simulink model "ENV_old"  (R2024b)
settings: Solver=FixedStepDiscrete  StartTime=0.0  StopTime=1  FixedStep=0.001  RelTol=1e-3  EnableMultiTasking=on
libraries: stm32blockslib x84, canmsglib x40, stm32f4xxblockslib x8, simulink x7
(part 2 of 4)

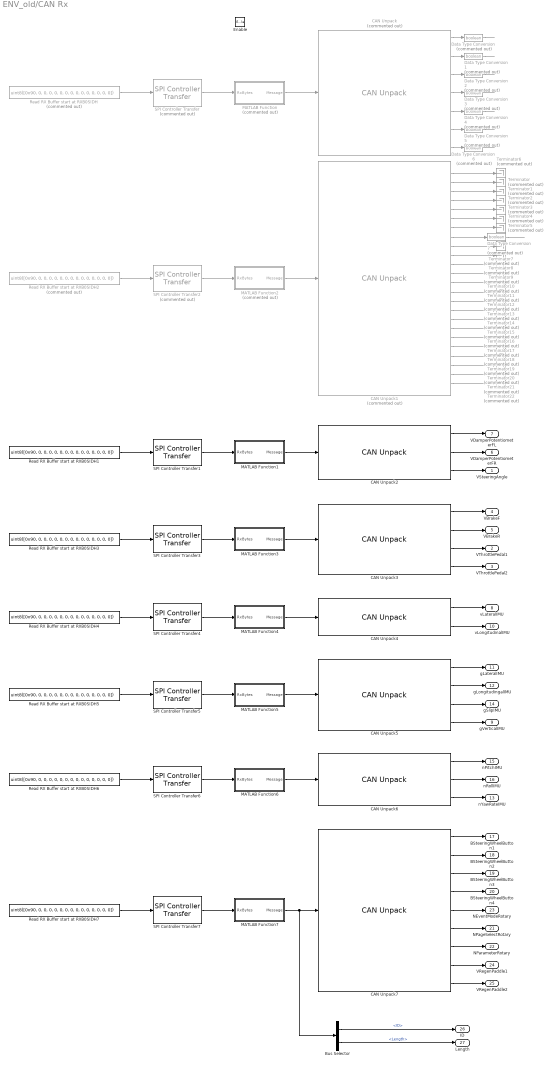
== system ENV_old/CAN Rx ==
  Enable : EnablePort
  Bus Selector : BusSelector  OutputSignals=ID,Length
  CAN Unpack : canmsglib/CAN Unpack  Commented=on  CANdbFile=C:\Users\oxbro\Documents\STM32CustomProjects\PDUSTM32\CAN3_28.06.26.dbc  MsgList=VCU_PDMReq  MsgName=VCU_PDMReq  MsgIDType=Standard (11-bit identifier)  MsgIdentifier=1539  MsgLength=7  SignalInfo={'BAccuFanOn','24','8','LE','unsigned','Standard','0','1','0','0','255';'BBrakeLight','0','8','LE','unsigned','Standard','0','1','0','0','255';'BInvLVOn','32','8','LE','unsigned','Standard','0','1','0','0','255';'BInverterFanOn','8','8','LE','unsigned','Standard','0','1','0','0','255';'BMotorRBHFanOn','16','8','LE','unsigned','Standard','0','8','0','0','255';'BPCComplete','40','8','LE','unsigned','Standard','0','1','0','0','255';'BReadyToDriveBuzzer','48','8','LE','unsigned','Standard','0','1','0','0','255'}  IDPort=off  TimestampPort=off  ErrorPort=off  RemotePort=off  LengthPort=off  StatusPort=off  ApplyMinMax=off
      settings: LibrarySourceBlock=stmutilitieslib/CAN Unpack  DataFormat=CANdb specified signals
  CAN Unpack1 : canmsglib/CAN Unpack  Commented=on  CANdbFile=C:\Users\will\Desktop\STM32Projects\PDUSTM32\CAN3_28.06.26.dbc  MsgList=VCU_1s_Frame4  MsgName=VCU_1s_Frame4  MsgIDType=Standard (11-bit identifier)  MsgIdentifier=419  MsgLength=6  SignalInfo={'BBMSP0A0COut','32','1','LE','unsigned','Standard','0','1','0','0','1';'BBMSP0A0EOut','33','1','LE','unsigned','Standard','0','1','0','0','1';'BBMSP0A10Out','34','1','LE','unsigned','Standard','0','1','0','0','1';'BBMSP0A80Out','35','1','LE','unsigned','Standard','0','1','0','0','1';'BBMSP0AC0Out','36','1','LE','unsigned','Standard','0','1','0','0','1';'BBMSP0AFAOut','37','1','LE','unsigned','Standard','0','1','0','0','1';'BBalancingOnOut','31','1','LE','unsigned','Standard','0','1','0','0','1';'BDrivetrainCoolingOn','1','1','LE','unsigned','Standard','0','1','0','0','1';'BDrivetrainCoolingOnEM','5','1','LE','unsigned','Standard','0','1','0','0','1';'BDrivetrainCoolingOnOW','6','2','LE','unsigned','Standard','0','1','-1','-1','2';'BEMSOn','13','1','LE','unsigned','Standard','0','1','0','0','1';'BEMSOnEM','14','1','LE','unsigned','Standard','0','1','0','0','1';'BEMSOnOW','15','2','LE','unsigned','Standard','0','1','-1','-1','2';'BSpinningModeOn','17','1','LE','unsigned','Standard','0','1','0','0','1';'BSpinningModeOnEM','18','1','LE','unsigned','Standard','0','1','0','0','1';'BSpinningModeOnOW','19','2','LE','unsigned','Standard','0','1','-1','-1','2';'BTCOn','9','1','LE','unsigned','Standard','0','1','0','0','1';'BTCOnEM','10','1','LE','unsigned','Standard','0','1','0','0','1';'BTCOnOW','11','2','LE','unsigned','Standard','0','1','-1','-1','2';'BTVOnEM','0','1','LE','unsigned','Standard','0','1','0','0','1';'BTVOnOW','2','2','LE','unsigned','Standard','0','1','-1','-1','2';'NEventMode','44','4','LE','unsigned','Standard','0','1','0','0','15';'NLap','38','6','LE','unsigned','Standard','0','1','0','0','63';'rSoE','21','10','LE','unsigned','Standard','0','0.1','0','0','102.3'}  IDPort=off  TimestampPort=off  ErrorPort=off  RemotePort=off  LengthPort=off  StatusPort=off  ApplyMinMax=off
      settings: LibrarySourceBlock=stmutilitieslib/CAN Unpack  DataFormat=CANdb specified signals
  CAN Unpack2 : canmsglib/CAN Unpack  CANdbFile=C:\Users\oxbro\Documents\STM32CustomProjects\VCUSTM32\OBR26_Controls_30-7-26\CAN\CAN3\CAN3_03.08.26.dbc  MsgList=DDU7_SteerDamper  MsgName=DDU7_SteerDamper  MsgIDType=Standard (11-bit identifier)  MsgIdentifier=257  MsgLength=8  SignalInfo={'VDamperPotentiometerFL','16','13','LE','unsigned','Standard','0','1','0','0','8191';'VDamperPotentiometerFR','29','13','LE','unsigned','Standard','0','1','0','0','8191';'VSteeringAngle','0','13','LE','unsigned','Standard','0','1','0','0','8191'}  IDPort=off  TimestampPort=off  ErrorPort=off  RemotePort=off  LengthPort=off  StatusPort=off  ApplyMinMax=off
      settings: LibrarySourceBlock=stmutilitieslib/CAN Unpack  DataFormat=CANdb specified signals
  CAN Unpack3 : canmsglib/CAN Unpack  CANdbFile=C:\Users\oxbro\Documents\STM32CustomProjects\VCUSTM32\OBR26_Controls_30-7-26\CAN\CAN3\CAN3_03.08.26.dbc  MsgList=DDU7_ThrBrake  MsgName=DDU7_ThrBrake  MsgIDType=Standard (11-bit identifier)  MsgIdentifier=256  MsgLength=8  SignalInfo={'VBrakeF','0','16','LE','unsigned','Standard','0','1','0','0','3276.75';'VBrakeR','16','16','LE','unsigned','Standard','0','1','0','0','65535';'VThrottlePedal1','32','16','LE','unsigned','Standard','0','1','0','0','65535';'VThrottlePedal2','48','16','LE','unsigned','Standard','0','1','0','0','65535'}  IDPort=off  TimestampPort=off  ErrorPort=off  RemotePort=off  LengthPort=off  StatusPort=off  ApplyMinMax=off
      settings: LibrarySourceBlock=stmutilitieslib/CAN Unpack  DataFormat=CANdb specified signals
  CAN Unpack4 : canmsglib/CAN Unpack  CANdbFile=C:\Users\oxbro\Documents\STM32CustomProjects\VCUSTM32\OBR26_Controls_30-7-26\CAN\CAN3\CAN3_03.08.26.dbc  MsgList=IMU_0x604  MsgName=IMU_0x604  MsgIDType=Standard (11-bit identifier)  MsgIdentifier=1540  MsgLength=8  SignalInfo={'vLateralIMU','16','16','LE','signed','Standard','0','0.01','0','-327.68','327.67';'vLongitudinalIMU','0','16','LE','signed','Standard','0','0.01','0','-327.68','327.67'}  IDPort=off  TimestampPort=off  ErrorPort=off  RemotePort=off  LengthPort=off  StatusPort=off  ApplyMinMax=off
      settings: LibrarySourceBlock=stmutilitieslib/CAN Unpack  DataFormat=CANdb specified signals
  CAN Unpack5 : canmsglib/CAN Unpack  CANdbFile=C:\Users\oxbro\Documents\STM32CustomProjects\VCUSTM32\OBR26_Controls_30-7-26\CAN\CAN3\CAN3_03.08.26.dbc  MsgList=IMU_0x606  MsgName=IMU_0x606  MsgIDType=Standard (11-bit identifier)  MsgIdentifier=1542  MsgLength=8  SignalInfo={'gLateralIMU','16','16','LE','signed','Standard','0','0.01','0','-327.68','327.67';'gLongitudinalIMU','0','16','LE','signed','Standard','0','0.01','0','-327.68','327.67';'gSlipIMU','48','16','LE','signed','Standard','0','0.01','0','-327.68','327.67';'gVerticalIMU','32','16','LE','signed','Standard','0','0.01','0','-327.68','327.67'}  IDPort=off  TimestampPort=off  ErrorPort=off  RemotePort=off  LengthPort=off  StatusPort=off  ApplyMinMax=off
      settings: LibrarySourceBlock=stmutilitieslib/CAN Unpack  DataFormat=CANdb specified signals
  CAN Unpack6 : canmsglib/CAN Unpack  CANdbFile=C:\Users\oxbro\Documents\STM32CustomProjects\VCUSTM32\OBR26_Controls_30-7-26\CAN\CAN3\CAN3_03.08.26.dbc  MsgList=IMU_0x609  MsgName=IMU_0x609  MsgIDType=Standard (11-bit identifier)  MsgIdentifier=1545  MsgLength=8  SignalInfo={'nPitchIMU','16','16','LE','signed','Standard','0','0.01','0','-327.68','327.67';'nRollIMU','0','16','LE','signed','Standard','0','0.01','0','-327.68','327.67';'nYawRateIMU','32','16','LE','signed','Standard','0','0.01','0','-327.68','327.67'}  IDPort=off  TimestampPort=off  ErrorPort=off  RemotePort=off  LengthPort=off  StatusPort=off  ApplyMinMax=off
      settings: LibrarySourceBlock=stmutilitieslib/CAN Unpack  DataFormat=CANdb specified signals
  CAN Unpack7 : canmsglib/CAN Unpack  CANdbFile=C:\Users\oxbro\Documents\STM32CustomProjects\VCUSTM32\OBR26_Controls_30-7-26\CAN\CAN3\CAN3_03.08.26.dbc  MsgList=STW_0x1FB  MsgName=STW_0x1FB  MsgIDType=Standard (11-bit identifier)  MsgIdentifier=507  MsgLength=6  SignalInfo={'BSteeringWheelButton1','0','1','LE','unsigned','Standard','0','1','0','0','1';'BSteeringWheelButton2','1','1','LE','unsigned','Standard','0','1','0','0','1';'BSteeringWheelButton3','2','1','LE','unsigned','Standard','0','1','0','0','1';'BSteeringWheelButton4','3','1','LE','unsigned','Standard','0','1','0','0','1';'NEventModeRotary','20','8','LE','unsigned','Standard','0','1','1','1','16';'NPageSelectRotary','4','8','LE','unsigned','Standard','0','1','1','1','16';'NParameterRotary','12','8','LE','unsigned','Standard','0','1','1','1','16';'VRegenPaddle1','28','8','LE','unsigned','Standard','0','0.0129','0','0','3.2895';'VRegenPaddle2','36','8','LE','unsigned','Standard','0','0.0129','0','0','3.2895'}  IDPort=off  TimestampPort=off  ErrorPort=off  RemotePort=off  LengthPort=off  StatusPort=off  ApplyMinMax=off
      settings: LibrarySourceBlock=stmutilitieslib/CAN Unpack  DataFormat=CANdb specified signals
  Data Type Conversion{,1..7} (8 alike) : DataTypeConversion  Commented=on  OutDataTypeStr=boolean  SaturateOnIntegerOverflow=off  RndMeth=Floor
  MATLAB Function : MATLAB Function  Commented=on  TreatAsAtomicUnit=on
  MATLAB Function1 : MATLAB Function  TreatAsAtomicUnit=on
  MATLAB Function2 : MATLAB Function  Commented=on  TreatAsAtomicUnit=on
  MATLAB Function3 : MATLAB Function  TreatAsAtomicUnit=on
  MATLAB Function4 : MATLAB Function  TreatAsAtomicUnit=on
  MATLAB Function5 : MATLAB Function  TreatAsAtomicUnit=on
  MATLAB Function6 : MATLAB Function  TreatAsAtomicUnit=on
  MATLAB Function7 : MATLAB Function  TreatAsAtomicUnit=on
  Read RX Buffer start at RXB0SIDH : Constant  Commented=on  Value=uint8([0x90, 0, 0, 0, 0, 0, 0, 0, 0, 0, 0, 0, 0, 0, 0])
  Read RX Buffer start at RXB0SIDH{1,3..7} (6 alike) : Constant  Value=uint8([0x90, 0, 0, 0, 0, 0, 0, 0, 0, 0, 0, 0, 0, 0, 0])
  Read RX Buffer start at RXB0SIDH2 : Constant  Commented=on  Value=uint8([0x90, 0, 0, 0, 0, 0, 0, 0, 0, 0, 0, 0, 0, 0, 0])
  SPI Controller Transfer : stm32blockslib/SPI Controller Transfer  Priority=1  Commented=on  SPIModuleSelect=SPI1  ClockPolarity=Low  ClockPhase=1 Edge  SPIModule=uint32(0)  Mode=Master  BusSpeed=uint32(1000000)  FirstBitToTransfer=Most significant bit (MSB)  ClockMode=0  BlockFunction=Transfer  EnableRegisterAddress=off  RegisterAddress=0  OutputDataType=uint8  OutputDataLength=1  OutputStatus=off  BlockingMode=on  Timeout=0.01  DataBits=8  UseCustomSSPin=Explicit GPIO calls  ActiveLowSSPin=Active low  Port_Select=GPIOA  Pin=1
      settings: LibrarySourceBlock=stm32h7xxblockslib/SPI Controller Transfer
  SPI Controller Transfer{1,3..7} (6 alike) : stm32blockslib/SPI Controller Transfer  Priority=1  SPIModuleSelect=SPI1  ClockPolarity=Low  ClockPhase=1 Edge  SPIModule=uint32(0)  Mode=Master  BusSpeed=uint32(1000000)  FirstBitToTransfer=Most significant bit (MSB)  ClockMode=0  BlockFunction=Transfer  EnableRegisterAddress=off  RegisterAddress=0  OutputDataType=uint8  OutputDataLength=1  OutputStatus=off  BlockingMode=on  Timeout=0.01  DataBits=8  UseCustomSSPin=Explicit GPIO calls  ActiveLowSSPin=Active low  Port_Select=GPIOA  Pin=1
      settings: LibrarySourceBlock=stm32h7xxblockslib/SPI Controller Transfer
  SPI Controller Transfer2 : stm32blockslib/SPI Controller Transfer  Priority=1  Commented=on  SPIModuleSelect=SPI1  ClockPolarity=Low  ClockPhase=1 Edge  SPIModule=uint32(0)  Mode=Master  BusSpeed=uint32(1000000)  FirstBitToTransfer=Most significant bit (MSB)  ClockMode=0  BlockFunction=Transfer  EnableRegisterAddress=off  RegisterAddress=0  OutputDataType=uint8  OutputDataLength=1  OutputStatus=off  BlockingMode=on  Timeout=0.01  DataBits=8  UseCustomSSPin=Explicit GPIO calls  ActiveLowSSPin=Active low  Port_Select=GPIOA  Pin=1
      settings: LibrarySourceBlock=stm32h7xxblockslib/SPI Controller Transfer
  Terminator{,1..22} (23 alike) : Terminator  Commented=on
  VSteeringAngle : Outport  OutDataTypeStr=double
  VThrottlePedal1 : Outport  Port=2  OutDataTypeStr=double
  VThrottlePedal2 : Outport  Port=3  OutDataTypeStr=double
  VBrakeF : Outport  Port=4  OutDataTypeStr=double
  VBrakeR : Outport  Port=5  OutDataTypeStr=double
  VDamperPotentiometerFR : Outport  Port=6  OutDataTypeStr=double
  VDamperPotentiometerFL : Outport  Port=7  OutDataTypeStr=double
  vLateralIMU : Outport  Port=8  OutDataTypeStr=double
  gVerticalIMU : Outport  Port=9  OutDataTypeStr=double
  vLongitudinalIMU : Outport  Port=10  OutDataTypeStr=double
  gLateralIMU : Outport  Port=11  OutDataTypeStr=double
  gLongitudingalIMU : Outport  Port=12  OutDataTypeStr=double
  nYawRateIMU : Outport  Port=13  OutDataTypeStr=double
  gSlipIMU : Outport  Port=14  OutDataTypeStr=double
  nPitchIMU : Outport  Port=15  OutDataTypeStr=double
  nRollIMU : Outport  Port=16  OutDataTypeStr=double
  BSteeringWheelButton1 : Outport  Port=17  OutDataTypeStr=boolean
  BSteeringWheelButton2 : Outport  Port=18  OutDataTypeStr=boolean
  BSteeringWheelButton3 : Outport  Port=19  OutDataTypeStr=boolean
  BSteeringWheelButton4 : Outport  Port=20  OutDataTypeStr=boolean
  NPageSelectRotary : Outport  Port=21  OutDataTypeStr=double
  NParameterRotary : Outport  Port=22  OutDataTypeStr=double
  NEventModeRotary : Outport  Port=23  OutDataTypeStr=double
  VRegenPaddle1 : Outport  Port=24  OutDataTypeStr=double
  VRegenPaddle2 : Outport  Port=25  OutDataTypeStr=double
  ID : Outport  Port=26
  Length : Outport  Port=27
  wires:
  Read RX Buffer start at RXB0SIDH/1 -> SPI Controller Transfer/1
  SPI Controller Transfer/1 -> MATLAB Function/1(RxBytes)
  MATLAB Function/1(Message) -> CAN Unpack/1
  CAN Unpack/1 -> Data Type Conversion/1
  CAN Unpack/2 -> Data Type Conversion1/1
  CAN Unpack1/2 -> Terminator/1
  CAN Unpack1/3 -> Terminator1/1
  CAN Unpack1/4 -> Terminator2/1
  CAN Unpack1/5 -> Terminator3/1
  CAN Unpack1/6 -> Terminator4/1
  CAN Unpack1/7 -> Terminator5/1
  CAN Unpack1/9 -> Terminator7/1
  CAN Unpack1/10 -> Terminator8/1
  CAN Unpack1/19 -> Terminator17/1
  CAN Unpack1/18 -> Terminator16/1
  CAN Unpack1/17 -> Terminator15/1
  CAN Unpack1/16 -> Terminator14/1
  CAN Unpack1/15 -> Terminator13/1
  CAN Unpack1/14 -> Terminator12/1
  CAN Unpack1/13 -> Terminator11/1
  CAN Unpack1/12 -> Terminator10/1
  CAN Unpack1/20 -> Terminator18/1
  CAN Unpack1/21 -> Terminator19/1
  CAN Unpack1/22 -> Terminator20/1
  CAN Unpack1/23 -> Terminator21/1
  CAN Unpack1/24 -> Terminator22/1
  CAN Unpack1/11 -> Terminator9/1
  CAN Unpack1/1 -> Terminator6/1
  Data Type Conversion/1 -> ?
  Data Type Conversion1/1 -> ?
  Data Type Conversion2/1 -> ?
  Data Type Conversion3/1 -> ?
  Data Type Conversion4/1 -> ?
  Data Type Conversion6/1 -> ?
  Data Type Conversion7/1 -> ?
  Data Type Conversion5/1 -> ?
  CAN Unpack1/8 -> Data Type Conversion7/1
  CAN Unpack/7 -> Data Type Conversion6/1
  Bus Selector/1 -> ID/1  "<ID>"
  Bus Selector/2 -> Length/1  "<Length>"
  Read RX Buffer start at RXB0SIDH2/1 -> SPI Controller Transfer2/1
  SPI Controller Transfer2/1 -> MATLAB Function2/1(RxBytes)
  MATLAB Function2/1(Message) -> CAN Unpack1/1
  CAN Unpack/3 -> Data Type Conversion2/1
  CAN Unpack/4 -> Data Type Conversion3/1
  CAN Unpack/5 -> Data Type Conversion4/1
  CAN Unpack/6 -> Data Type Conversion5/1
  CAN Unpack4/1 -> vLateralIMU/1
  CAN Unpack7/5 -> NEventModeRotary/1
  CAN Unpack7/3 -> BSteeringWheelButton3/1
  CAN Unpack2/1 -> VDamperPotentiometerFL/1
  CAN Unpack2/2 -> VDamperPotentiometerFR/1
  CAN Unpack5/4 -> gVerticalIMU/1
  CAN Unpack3/3 -> VThrottlePedal1/1
  CAN Unpack2/3 -> VSteeringAngle/1
  CAN Unpack6/2 -> nRollIMU/1
  CAN Unpack7/6 -> NPageSelectRotary/1
  CAN Unpack7/1 -> BSteeringWheelButton1/1
  CAN Unpack6/3 -> nYawRateIMU/1
  CAN Unpack3/1 -> VBrakeF/1
  CAN Unpack5/2 -> gLongitudingalIMU/1
  CAN Unpack7/9 -> VRegenPaddle2/1
  CAN Unpack7/7 -> NParameterRotary/1
  CAN Unpack7/2 -> BSteeringWheelButton2/1
  CAN Unpack3/4 -> VThrottlePedal2/1
  CAN Unpack3/2 -> VBrakeR/1
  CAN Unpack7/8 -> VRegenPaddle1/1
  CAN Unpack6/1 -> nPitchIMU/1
  CAN Unpack5/3 -> gSlipIMU/1
  CAN Unpack7/4 -> BSteeringWheelButton4/1
  CAN Unpack4/2 -> vLongitudinalIMU/1
  CAN Unpack5/1 -> gLateralIMU/1
  Read RX Buffer start at RXB0SIDH1/1 -> SPI Controller Transfer1/1
  SPI Controller Transfer1/1 -> MATLAB Function1/1(RxBytes)
  MATLAB Function1/1(Message) -> CAN Unpack2/1
  MATLAB Function3/1(Message) -> CAN Unpack3/1
  Read RX Buffer start at RXB0SIDH3/1 -> SPI Controller Transfer3/1
  SPI Controller Transfer3/1 -> MATLAB Function3/1(RxBytes)
  MATLAB Function4/1(Message) -> CAN Unpack4/1
  Read RX Buffer start at RXB0SIDH4/1 -> SPI Controller Transfer4/1
  SPI Controller Transfer4/1 -> MATLAB Function4/1(RxBytes)
  Read RX Buffer start at RXB0SIDH5/1 -> SPI Controller Transfer5/1
  SPI Controller Transfer5/1 -> MATLAB Function5/1(RxBytes)
  MATLAB Function5/1(Message) -> CAN Unpack5/1
  Read RX Buffer start at RXB0SIDH6/1 -> SPI Controller Transfer6/1
  SPI Controller Transfer6/1 -> MATLAB Function6/1(RxBytes)
  MATLAB Function6/1(Message) -> CAN Unpack6/1
  Read RX Buffer start at RXB0SIDH7/1 -> SPI Controller Transfer7/1
  SPI Controller Transfer7/1 -> MATLAB Function7/1(RxBytes)
  MATLAB Function7/1(Message) -> Bus Selector/1, CAN Unpack7/1

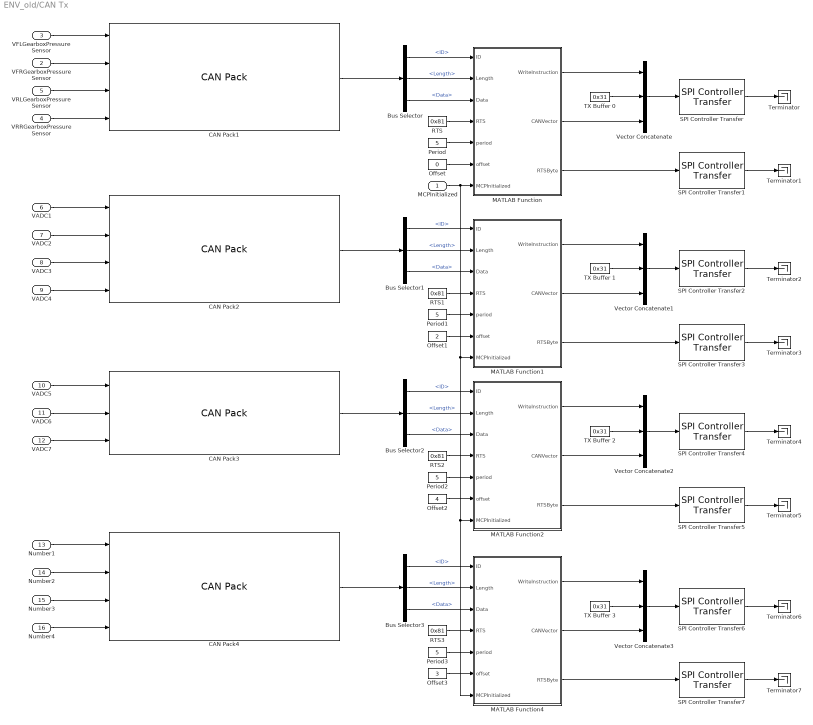
== system ENV_old/CAN Tx ==
  MCPInitialized : Inport
  VFRGearboxPressureSensor : Inport  Port=2
  VFLGearboxPressureSensor : Inport  Port=3
  VRRGearboxPressureSensor : Inport  Port=4
  VRLGearboxPressureSensor : Inport  Port=5
  VADC1 : Inport  Port=6
  VADC2 : Inport  Port=7
  VADC3 : Inport  Port=8
  VADC4 : Inport  Port=9
  VADC5 : Inport  Port=10
  VADC6 : Inport  Port=11
  VADC7 : Inport  Port=12
  Number1 : Inport  Port=13
  Number2 : Inport  Port=14
  Number3 : Inport  Port=15
  Number4 : Inport  Port=16
  Bus Selector{,1..3} (4 alike) : BusSelector  OutputSignals=ID,Length,Data
  CAN Pack1 : canmsglib/CAN Pack  CANdbFile=C:\Users\oxbro\Documents\STM32CustomProjects\PDUSTM32\ADCTest.dbc  MsgList=GearboxPressures  MsgName=GearboxPressures  MsgIDType=Standard (11-bit identifier)  MsgIdentifier=105  CANIDInput=off  MsgLength=8  Remote=off  ApplyMinMax=off  BusOutput=on  SignalInfo={'VFLGearboxPressureSensor','0','12','LE','unsigned','Standard','0','0.0012211','0','0','5.0004';'VFRGearboxPressureSensor','16','12','LE','unsigned','Standard','0','0.0012211','0','0','5.0004';'VRLGearboxPressureSensor','32','12','LE','unsigned','Standard','0','0.0012211','0','0','5.0004';'VRRGearboxPressureSensor','48','12','LE','unsigned','Standard','0','0.0012211','0','0','5.0004'}
      settings: LibrarySourceBlock=stmutilitieslib/CAN Pack  DataFormat=CANdb specified signals
  CAN Pack2 : canmsglib/CAN Pack  CANdbFile=C:\Users\oxbro\Documents\STM32CustomProjects\PDUSTM32\ADCTest.dbc  MsgList=ADCs1  MsgName=ADCs1  MsgIDType=Standard (11-bit identifier)  MsgIdentifier=5  CANIDInput=off  MsgLength=8  Remote=off  ApplyMinMax=off  BusOutput=on  SignalInfo={'VADC1','0','16','LE','unsigned','Standard','0','5.04e-05','0','0','3.303';'VADC2','16','16','LE','unsigned','Standard','0','5.04e-05','0','0','3.303';'VADC3','32','16','LE','unsigned','Standard','0','5.04e-05','0','0','3.303';'VADC4','48','16','LE','unsigned','Standard','0','5.04e-05','0','0','3.303'}
      settings: LibrarySourceBlock=stmutilitieslib/CAN Pack  DataFormat=CANdb specified signals
  CAN Pack3 : canmsglib/CAN Pack  CANdbFile=C:\Users\oxbro\Documents\STM32CustomProjects\PDUSTM32\ADCTest.dbc  MsgList=ADCs2  MsgName=ADCs2  MsgIDType=Standard (11-bit identifier)  MsgIdentifier=66  CANIDInput=off  MsgLength=6  Remote=off  ApplyMinMax=off  BusOutput=on  SignalInfo={'VADC5','0','16','LE','unsigned','Standard','0','5.04e-05','0','0','3.303';'VADC6','16','16','LE','unsigned','Standard','0','5.04e-05','0','0','3.303';'VLVSystem','32','16','LE','unsigned','Standard','0','0.00046327','0','0','30.3604'}
      settings: LibrarySourceBlock=stmutilitieslib/CAN Pack  DataFormat=CANdb specified signals
  CAN Pack4 : canmsglib/CAN Pack  CANdbFile=C:\Users\oxbro\Documents\STM32CustomProjects\PDUSTM32\ADCTest.dbc  MsgList=Numbers  MsgName=Numbers  MsgIDType=Standard (11-bit identifier)  MsgIdentifier=0  CANIDInput=off  MsgLength=8  Remote=off  ApplyMinMax=off  BusOutput=on  SignalInfo={'Number1','0','16','LE','signed','Standard','0','1','0','-32768','32767';'Number2','16','16','LE','signed','Standard','0','1','0','-32768','32767';'Number3','32','16','LE','signed','Standard','0','1','0','-32768','32767';'Number4','48','16','LE','signed','Standard','0','1','0','-32768','32767'}
      settings: LibrarySourceBlock=stmutilitieslib/CAN Pack  DataFormat=CANdb specified signals
  MATLAB Function : MATLAB Function  TreatAsAtomicUnit=on
  MATLAB Function1 : MATLAB Function  TreatAsAtomicUnit=on
  MATLAB Function2 : MATLAB Function  TreatAsAtomicUnit=on
  MATLAB Function4 : MATLAB Function  TreatAsAtomicUnit=on
  Offset : Constant  Value=0  OutDataTypeStr=uint16  SampleTime=-1
  Offset1 : Constant  Value=2  OutDataTypeStr=uint16  SampleTime=-1
  Offset2 : Constant  Value=4  OutDataTypeStr=uint16  SampleTime=-1
  Offset3 : Constant  Value=3  OutDataTypeStr=uint16  SampleTime=-1
  Period{,1..3} (4 alike) : Constant  Value=5  OutDataTypeStr=uint16  SampleTime=-1
  RTS{,1..3} (4 alike) : Constant  Value=0x81  OutDataTypeStr=uint8  SampleTime=-1
  SPI Controller Transfer{,2,4,6} (4 alike) : stm32blockslib/SPI Controller Transfer  Priority=1  SPIModuleSelect=SPI1  ClockPolarity=Low  ClockPhase=1 Edge  SPIModule=uint32(0)  Mode=Master  BusSpeed=uint32(1000000)  FirstBitToTransfer=Most significant bit (MSB)  ClockMode=0  BlockFunction=Transfer  EnableRegisterAddress=off  RegisterAddress=0  OutputDataType=uint8  OutputDataLength=1  OutputStatus=off  BlockingMode=off  Timeout=0.01  DataBits=8  UseCustomSSPin=Explicit GPIO calls  ActiveLowSSPin=Active low  Port_Select=GPIOA  Pin=1
      settings: LibrarySourceBlock=stm32h7xxblockslib/SPI Controller Transfer
  SPI Controller Transfer{1,3,5,7} (4 alike) : stm32blockslib/SPI Controller Transfer  Priority=2  SPIModuleSelect=SPI1  ClockPolarity=Low  ClockPhase=1 Edge  SPIModule=uint32(0)  Mode=Master  BusSpeed=uint32(1000000)  FirstBitToTransfer=Most significant bit (MSB)  ClockMode=0  BlockFunction=Transfer  EnableRegisterAddress=off  RegisterAddress=0  OutputDataType=uint8  OutputDataLength=1  OutputStatus=off  BlockingMode=off  Timeout=0.01  DataBits=8  UseCustomSSPin=Explicit GPIO calls  ActiveLowSSPin=Active low  Port_Select=GPIOA  Pin=1
      settings: LibrarySourceBlock=stm32h7xxblockslib/SPI Controller Transfer
  TX Buffer {0..3} (4 alike) : Constant  Value=0x31  OutDataTypeStr=uint8  SampleTime=-1
  Terminator{,1..7} (8 alike) : Terminator
  Vector Concatenate{,1..3} (4 alike) : Concatenate  NumInputs=3
  wires:
  SPI Controller Transfer/1 -> Terminator/1
  MATLAB Function/1(WriteInstruction) -> Vector Concatenate/1
  RTS/1 -> MATLAB Function/4(RTS)
  MATLAB Function/2(CANVector) -> Vector Concatenate/3
  SPI Controller Transfer1/1 -> Terminator1/1
  Bus Selector/1 -> MATLAB Function/1(ID)  "<ID>"
  Vector Concatenate/1 -> SPI Controller Transfer/1
  TX Buffer 0/1 -> Vector Concatenate/2
  MATLAB Function/3(RTSByte) -> SPI Controller Transfer1/1
  Bus Selector/2 -> MATLAB Function/2(Length)  "<Length>"
  Bus Selector/3 -> MATLAB Function/3(Data)  "<Data>"
  CAN Pack1/1 -> Bus Selector/1
  Period/1 -> MATLAB Function/5(period)
  Offset/1 -> MATLAB Function/6(offset)
  VRLGearboxPressureSensor/1 -> CAN Pack1/3
  VRRGearboxPressureSensor/1 -> CAN Pack1/4
  VFRGearboxPressureSensor/1 -> CAN Pack1/2
  VFLGearboxPressureSensor/1 -> CAN Pack1/1
  SPI Controller Transfer2/1 -> Terminator2/1
  SPI Controller Transfer3/1 -> Terminator3/1
  RTS1/1 -> MATLAB Function1/4(RTS)
  MATLAB Function1/2(CANVector) -> Vector Concatenate1/3
  Bus Selector1/3 -> MATLAB Function1/3(Data)  "<Data>"
  Period1/1 -> MATLAB Function1/5(period)
  Bus Selector1/2 -> MATLAB Function1/2(Length)  "<Length>"
  Offset1/1 -> MATLAB Function1/6(offset)
  CAN Pack2/1 -> Bus Selector1/1
  Bus Selector1/1 -> MATLAB Function1/1(ID)  "<ID>"
  MATLAB Function1/3(RTSByte) -> SPI Controller Transfer3/1
  Vector Concatenate1/1 -> SPI Controller Transfer2/1
  MATLAB Function1/1(WriteInstruction) -> Vector Concatenate1/1
  TX Buffer 1/1 -> Vector Concatenate1/2
  SPI Controller Transfer4/1 -> Terminator4/1
  SPI Controller Transfer5/1 -> Terminator5/1
  RTS2/1 -> MATLAB Function2/4(RTS)
  MATLAB Function2/2(CANVector) -> Vector Concatenate2/3
  Bus Selector2/3 -> MATLAB Function2/3(Data)  "<Data>"
  Period2/1 -> MATLAB Function2/5(period)
  Bus Selector2/2 -> MATLAB Function2/2(Length)  "<Length>"
  Offset2/1 -> MATLAB Function2/6(offset)
  CAN Pack3/1 -> Bus Selector2/1
  Bus Selector2/1 -> MATLAB Function2/1(ID)  "<ID>"
  MATLAB Function2/3(RTSByte) -> SPI Controller Transfer5/1
  Vector Concatenate2/1 -> SPI Controller Transfer4/1
  MATLAB Function2/1(WriteInstruction) -> Vector Concatenate2/1
  TX Buffer 2/1 -> Vector Concatenate2/2
  VADC1/1 -> CAN Pack2/1
  VADC2/1 -> CAN Pack2/2
  VADC3/1 -> CAN Pack2/3
  VADC4/1 -> CAN Pack2/4
  VADC5/1 -> CAN Pack3/1
  VADC6/1 -> CAN Pack3/2
  VADC7/1 -> CAN Pack3/3
  Period3/1 -> MATLAB Function4/5(period)
  Vector Concatenate3/1 -> SPI Controller Transfer6/1
  Offset3/1 -> MATLAB Function4/6(offset)
  Number1/1 -> CAN Pack4/1
  MATLAB Function4/3(RTSByte) -> SPI Controller Transfer7/1
  Number4/1 -> CAN Pack4/4
  MCPInitialized/1 -> MATLAB Function4/7(MCPInitialized), MATLAB Function2/7(MCPInitialized), MATLAB Function1/7(MCPInitialized), MATLAB Function/7(MCPInitialized)
  MATLAB Function4/2(CANVector) -> Vector Concatenate3/3
  Number3/1 -> CAN Pack4/3
  Bus Selector3/3 -> MATLAB Function4/3(Data)  "<Data>"
  Number2/1 -> CAN Pack4/2
  CAN Pack4/1 -> Bus Selector3/1
  Bus Selector3/1 -> MATLAB Function4/1(ID)  "<ID>"
  MATLAB Function4/1(WriteInstruction) -> Vector Concatenate3/1
  TX Buffer 3/1 -> Vector Concatenate3/2
  SPI Controller Transfer6/1 -> Terminator6/1
  SPI Controller Transfer7/1 -> Terminator7/1
  Bus Selector3/2 -> MATLAB Function4/2(Length)  "<Length>"
  RTS3/1 -> MATLAB Function4/4(RTS)

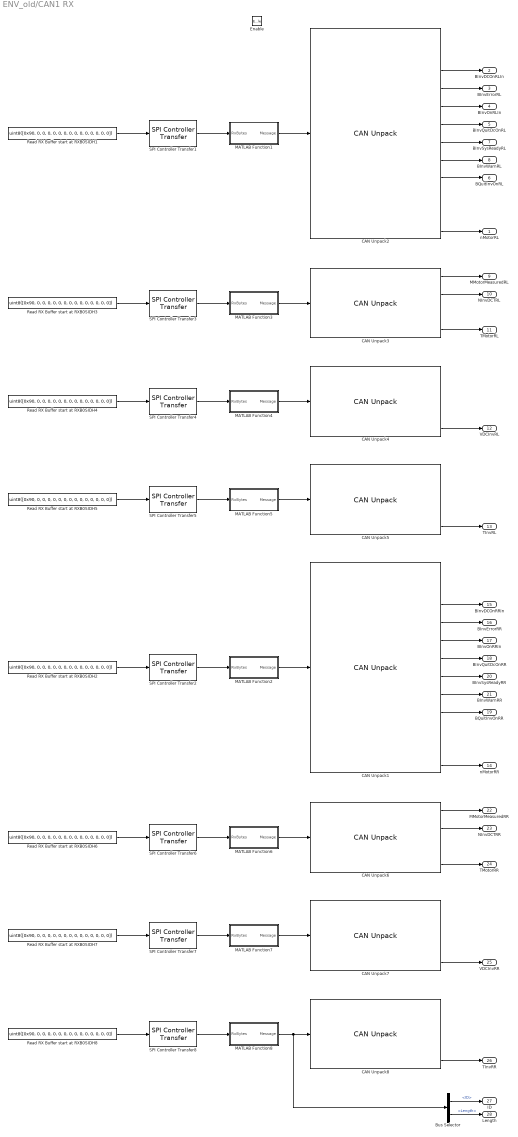
== system ENV_old/CAN1 RX ==
  Enable : EnablePort
  Bus Selector : BusSelector  OutputSignals=ID,Length
  CAN Unpack1 : canmsglib/CAN Unpack  CANdbFile=C:\Users\Will\Desktop\OBR\Embedded\VCUSTM32\Controls\CAN\Inverters\26.06.18_CAN1.dbc  MsgList=INV3_Send_1  MsgName=INV3_Send_1  MsgIDType=Standard (11-bit identifier)  MsgIdentifier=644  MsgLength=8  SignalInfo={'AMK_bDerating','47','1','LE','unsigned','Standard','0','1','0','0','1';'AMK_bReserve','32','8','LE','signed','Standard','0','1','0','-128','127';'BInvDCOnRRIn','44','1','LE','unsigned','Standard','0','1','0','0','1';'BInvErrorRR','41','1','LE','unsigned','Standard','0','1','0','0','1';'BInvOnRRIn','46','1','LE','unsigned','Standard','0','1','0','0','1';'BInvQuitDcOnRR','43','1','LE','unsigned','Standard','0','1','0','0','1';'BInvSysReadyRR','40','1','LE','unsigned','Standard','0','1','0','0','1';'BInvWarnRR','42','1','LE','unsigned','Standard','0','1','0','0','1';'BQuitInvOnRR','45','1','LE','unsigned','Standard','0','1','0','0','1';'Checksum','16','16','LE','unsigned','Standard','0','1','0','0','65535';'Message_Counter','0','16','LE','unsigned','Standard','0','1','0','0','65535';'nMotorRR','48','16','LE','signed','Standard','0','1','0','-32768','32767'}  IDPort=off  TimestampPort=off  ErrorPort=off  RemotePort=off  LengthPort=off  StatusPort=off  ApplyMinMax=off
      settings: LibrarySourceBlock=stmutilitieslib/CAN Unpack  DataFormat=CANdb specified signals
  CAN Unpack2 : canmsglib/CAN Unpack  CANdbFile=C:\Users\Will\Desktop\OBR\Embedded\VCUSTM32\Controls\CAN\Inverters\26.06.18_CAN1.dbc  MsgList=INV1_Send_1  MsgName=INV1_Send_1  MsgIDType=Standard (11-bit identifier)  MsgIdentifier=643  MsgLength=8  SignalInfo={'AMK_bDerating','47','1','LE','unsigned','Standard','0','1','0','0','1';'AMK_bReserve','32','8','LE','signed','Standard','0','1','0','-128','127';'BInvDCOnRLIn','44','1','LE','unsigned','Standard','0','1','0','0','1';'BInvErrorRL','41','1','LE','unsigned','Standard','0','1','0','0','1';'BInvOnRLIn','46','1','LE','unsigned','Standard','0','1','0','0','1';'BInvQuitDcOnRL','43','1','LE','unsigned','Standard','0','1','0','0','1';'BInvSysReadyRL','40','1','LE','unsigned','Standard','0','1','0','0','1';'BInvWarnRL','42','1','LE','unsigned','Standard','0','1','0','0','1';'BQuitInvOnRL','45','1','LE','unsigned','Standard','0','1','0','0','1';'Checksum','16','16','LE','unsigned','Standard','0','1','0','0','65535';'Message_Counter','0','16','LE','unsigned','Standard','0','1','0','0','65535';'nMotorRL','48','16','LE','signed','Standard','0','1','0','-32768','32767'}  IDPort=off  TimestampPort=off  ErrorPort=off  RemotePort=off  LengthPort=off  StatusPort=off  ApplyMinMax=off
      settings: LibrarySourceBlock=stmutilitieslib/CAN Unpack  DataFormat=CANdb specified signals
  CAN Unpack3 : canmsglib/CAN Unpack  CANdbFile=C:\Users\Will\Desktop\OBR\Embedded\VCUSTM32\Controls\CAN\Inverters\26.06.18_CAN1.dbc  MsgList=INV1_Send_2  MsgName=INV1_Send_2  MsgIDType=Standard (11-bit identifier)  MsgIdentifier=645  MsgLength=8  SignalInfo={'MMotorMeasuredRL','16','16','LE','signed','Standard','0','1','0','-32768','32767';'NInvDTCRL','32','16','LE','signed','Standard','0','1','0','-32768','32767';'NInvErrorInfoRL1','48','16','LE','signed','Standard','0','1','0','-32768','32767';'TMotorRL','0','16','LE','signed','Standard','0','0.1','0','-3276.8','3276.7'}  IDPort=off  TimestampPort=off  ErrorPort=off  RemotePort=off  LengthPort=off  StatusPort=off  ApplyMinMax=off
      settings: LibrarySourceBlock=stmutilitieslib/CAN Unpack  DataFormat=CANdb specified signals
  CAN Unpack4 : canmsglib/CAN Unpack  CANdbFile=C:\Users\Will\Desktop\OBR\Embedded\VCUSTM32\Controls\CAN\Inverters\26.06.18_CAN1.dbc  MsgList=INV1_Send_3  MsgName=INV1_Send_3  MsgIDType=Standard (11-bit identifier)  MsgIdentifier=647  MsgLength=8  SignalInfo={'NInvErrorInfoRL2','0','16','LE','signed','Standard','0','1','0','-32768','32767';'NInvErrorInfoRL3','16','16','LE','signed','Standard','0','1','0','-32768','32767';'Raw_Torque_Current','32','16','LE','signed','Standard','0','1','0','-32768','32767';'VDCInvRL','48','16','LE','signed','Standard','0','1','0','-32768','32767'}  IDPort=off  TimestampPort=off  ErrorPort=off  RemotePort=off  LengthPort=off  StatusPort=off  ApplyMinMax=off
      settings: LibrarySourceBlock=stmutilitieslib/CAN Unpack  DataFormat=CANdb specified signals
  CAN Unpack5 : canmsglib/CAN Unpack  CANdbFile=C:\Users\Will\Desktop\OBR\Embedded\VCUSTM32\Controls\CAN\Inverters\26.06.18_CAN1.dbc  MsgList=INV1_Send_4  MsgName=INV1_Send_4  MsgIDType=Standard (11-bit identifier)  MsgIdentifier=649  MsgLength=8  SignalInfo={'Converter_Peak_Current','32','16','LE','signed','Standard','0','1','0','-32768','32767';'Motor_Nomial_Current_IN','48','16','LE','signed','Standard','0','1','0','-32768','32767';'Motor_Peak_Current','16','16','LE','signed','Standard','0','1','0','-32768','32767';'TInvRL','0','16','LE','signed','Standard','0','0.1','0','-3276.8','3276.7'}  IDPort=off  TimestampPort=off  ErrorPort=off  RemotePort=off  LengthPort=off  StatusPort=off  ApplyMinMax=off
      settings: LibrarySourceBlock=stmutilitieslib/CAN Unpack  DataFormat=CANdb specified signals
  CAN Unpack6 : canmsglib/CAN Unpack  CANdbFile=C:\Users\Will\Desktop\OBR\Embedded\VCUSTM32\Controls\CAN\Inverters\26.06.18_CAN1.dbc  MsgList=INV3_Send_2  MsgName=INV3_Send_2  MsgIDType=Standard (11-bit identifier)  MsgIdentifier=646  MsgLength=8  SignalInfo={'MMotorMeasuredRR','16','16','LE','signed','Standard','0','1','0','-32768','32767';'NInvDTCRR','32','16','LE','signed','Standard','0','1','0','-32768','32767';'NInvErrorInfoRR1','48','16','LE','signed','Standard','0','1','0','-32768','32767';'TMotorRR','0','16','LE','signed','Standard','0','0.1','0','-3276.8','3276.7'}  IDPort=off  TimestampPort=off  ErrorPort=off  RemotePort=off  LengthPort=off  StatusPort=off  ApplyMinMax=off
      settings: LibrarySourceBlock=stmutilitieslib/CAN Unpack  DataFormat=CANdb specified signals
  CAN Unpack7 : canmsglib/CAN Unpack  CANdbFile=C:\Users\Will\Desktop\OBR\Embedded\VCUSTM32\Controls\CAN\Inverters\26.06.18_CAN1.dbc  MsgList=INV3_Send_3  MsgName=INV3_Send_3  MsgIDType=Standard (11-bit identifier)  MsgIdentifier=648  MsgLength=8  SignalInfo={'NInvErrorInfoRR2','0','16','LE','signed','Standard','0','1','0','-32768','32767';'NInvErrorInfoRR3','16','16','LE','signed','Standard','0','1','0','-32768','32767';'Raw_Torque_Current','32','16','LE','signed','Standard','0','1','0','-32768','32767';'VDCInvRR','48','16','LE','signed','Standard','0','1','0','-32768','32767'}  IDPort=off  TimestampPort=off  ErrorPort=off  RemotePort=off  LengthPort=off  StatusPort=off  ApplyMinMax=off
      settings: LibrarySourceBlock=stmutilitieslib/CAN Unpack  DataFormat=CANdb specified signals
  CAN Unpack8 : canmsglib/CAN Unpack  CANdbFile=C:\Users\Will\Desktop\OBR\Embedded\VCUSTM32\Controls\CAN\Inverters\26.06.18_CAN1.dbc  MsgList=INV3_Send_4  MsgName=INV3_Send_4  MsgIDType=Standard (11-bit identifier)  MsgIdentifier=656  MsgLength=8  SignalInfo={'Converter_Peak_Current','32','16','LE','signed','Standard','0','1','0','-32768','32767';'Motor_Nomial_Current_IN','48','16','LE','signed','Standard','0','1','0','-32768','32767';'Motor_Peak_Current','16','16','LE','signed','Standard','0','1','0','-32768','32767';'TInvRR','0','16','LE','signed','Standard','0','0.1','0','-3276.8','3276.7'}  IDPort=off  TimestampPort=off  ErrorPort=off  RemotePort=off  LengthPort=off  StatusPort=off  ApplyMinMax=off
      settings: LibrarySourceBlock=stmutilitieslib/CAN Unpack  DataFormat=CANdb specified signals
  MATLAB Function1 : MATLAB Function  TreatAsAtomicUnit=on
  MATLAB Function2 : MATLAB Function  TreatAsAtomicUnit=on
  MATLAB Function3 : MATLAB Function  TreatAsAtomicUnit=on
  MATLAB Function4 : MATLAB Function  TreatAsAtomicUnit=on
  MATLAB Function5 : MATLAB Function  TreatAsAtomicUnit=on
  MATLAB Function6 : MATLAB Function  TreatAsAtomicUnit=on
  MATLAB Function7 : MATLAB Function  TreatAsAtomicUnit=on
  MATLAB Function8 : MATLAB Function  TreatAsAtomicUnit=on
  Read RX Buffer start at RXB0SIDH{1..8} (8 alike) : Constant  Value=uint8([0x90, 0, 0, 0, 0, 0, 0, 0, 0, 0, 0, 0, 0, 0, 0])
  SPI Controller Transfer{1..8} (8 alike) : stm32blockslib/SPI Controller Transfer  Priority=1  SPIModuleSelect=SPI1  ClockPolarity=Low  ClockPhase=1 Edge  SPIModule=uint32(0)  Mode=Master  BusSpeed=uint32(1000000)  FirstBitToTransfer=Most significant bit (MSB)  ClockMode=0  BlockFunction=Transfer  EnableRegisterAddress=off  RegisterAddress=0  OutputDataType=uint8  OutputDataLength=1  OutputStatus=off  BlockingMode=on  Timeout=0.01  DataBits=8  UseCustomSSPin=Explicit GPIO calls  ActiveLowSSPin=Active low  Port_Select=GPIOB  Pin=1
      settings: LibrarySourceBlock=stm32h7xxblockslib/SPI Controller Transfer
  nMotorRL : Outport  OutDataTypeStr=double
  BInvDCOnRLIn : Outport  Port=2  OutDataTypeStr=boolean
  BInvErrorRL : Outport  Port=3  OutDataTypeStr=boolean
  BInvOnRLIn : Outport  Port=4  OutDataTypeStr=boolean
  BInvQuitDcOnRL : Outport  Port=5  OutDataTypeStr=boolean
  BQuitInvOnRL : Outport  Port=6  OutDataTypeStr=boolean
  BInvSysReadyRL : Outport  Port=7  OutDataTypeStr=boolean
  BInvWarnRL : Outport  Port=8  OutDataTypeStr=boolean
  MMotorMeasuredRL : Outport  Port=9  OutDataTypeStr=double
  NInvDCTRL : Outport  Port=10  OutDataTypeStr=double
  TMotorRL : Outport  Port=11  OutDataTypeStr=double
  VDCInvRL : Outport  Port=12  OutDataTypeStr=double
  TInvRL : Outport  Port=13  OutDataTypeStr=double
  nMotorRR : Outport  Port=14  OutDataTypeStr=double
  BInvDCOnRRIn : Outport  Port=15  OutDataTypeStr=boolean
  BInvErrorRR : Outport  Port=16  OutDataTypeStr=boolean
  BInvOnRRIn : Outport  Port=17  OutDataTypeStr=boolean
  BInvQuitDcOnRR : Outport  Port=18  OutDataTypeStr=boolean
  BQuitInvOnRR : Outport  Port=19  OutDataTypeStr=boolean
  BInvSysReadyRR : Outport  Port=20  OutDataTypeStr=boolean
  BInvWarnRR : Outport  Port=21  OutDataTypeStr=boolean
  MMotorMeasuredRR : Outport  Port=22  OutDataTypeStr=double
  NInvDCTRR : Outport  Port=23  OutDataTypeStr=double
  TMotorRR : Outport  Port=24  OutDataTypeStr=double
  VDCInvRR : Outport  Port=25  OutDataTypeStr=double
  TInvRR : Outport  Port=26  OutDataTypeStr=double
  ID : Outport  Port=27
  Length : Outport  Port=28
  wires:
  Read RX Buffer start at RXB0SIDH1/1 -> SPI Controller Transfer1/1
  SPI Controller Transfer1/1 -> MATLAB Function1/1(RxBytes)
  MATLAB Function1/1(Message) -> CAN Unpack2/1
  CAN Unpack2/3 -> BInvDCOnRLIn/1
  CAN Unpack2/4 -> BInvErrorRL/1
  CAN Unpack2/5 -> BInvOnRLIn/1
  CAN Unpack2/6 -> BInvQuitDcOnRL/1
  CAN Unpack2/9 -> BQuitInvOnRL/1
  CAN Unpack2/8 -> BInvWarnRL/1
  CAN Unpack2/7 -> BInvSysReadyRL/1
  CAN Unpack2/12 -> nMotorRL/1
  CAN Unpack3/4 -> TMotorRL/1
  MATLAB Function3/1(Message) -> CAN Unpack3/1
  SPI Controller Transfer3/1 -> MATLAB Function3/1(RxBytes)
  Read RX Buffer start at RXB0SIDH3/1 -> SPI Controller Transfer3/1
  CAN Unpack3/1 -> MMotorMeasuredRL/1
  CAN Unpack3/2 -> NInvDCTRL/1
  CAN Unpack4/4 -> VDCInvRL/1
  SPI Controller Transfer4/1 -> MATLAB Function4/1(RxBytes)
  MATLAB Function4/1(Message) -> CAN Unpack4/1
  Read RX Buffer start at RXB0SIDH4/1 -> SPI Controller Transfer4/1
  SPI Controller Transfer5/1 -> MATLAB Function5/1(RxBytes)
  CAN Unpack5/4 -> TInvRL/1
  Read RX Buffer start at RXB0SIDH5/1 -> SPI Controller Transfer5/1
  MATLAB Function5/1(Message) -> CAN Unpack5/1
  MATLAB Function8/1(Message) -> CAN Unpack8/1, Bus Selector/1
  Bus Selector/2 -> Length/1  "<Length>"
  Bus Selector/1 -> ID/1  "<ID>"
  CAN Unpack1/6 -> BInvQuitDcOnRR/1
  CAN Unpack1/3 -> BInvDCOnRRIn/1
  CAN Unpack6/4 -> TMotorRR/1
  CAN Unpack1/5 -> BInvOnRRIn/1
  SPI Controller Transfer2/1 -> MATLAB Function2/1(RxBytes)
  MATLAB Function2/1(Message) -> CAN Unpack1/1
  SPI Controller Transfer8/1 -> MATLAB Function8/1(RxBytes)
  CAN Unpack1/8 -> BInvWarnRR/1
  CAN Unpack6/1 -> MMotorMeasuredRR/1
  CAN Unpack1/12 -> nMotorRR/1
  CAN Unpack1/4 -> BInvErrorRR/1
  CAN Unpack1/7 -> BInvSysReadyRR/1
  CAN Unpack1/9 -> BQuitInvOnRR/1
  Read RX Buffer start at RXB0SIDH2/1 -> SPI Controller Transfer2/1
  SPI Controller Transfer7/1 -> MATLAB Function7/1(RxBytes)
  Read RX Buffer start at RXB0SIDH8/1 -> SPI Controller Transfer8/1
  MATLAB Function6/1(Message) -> CAN Unpack6/1
  Read RX Buffer start at RXB0SIDH7/1 -> SPI Controller Transfer7/1
  CAN Unpack6/2 -> NInvDCTRR/1
  SPI Controller Transfer6/1 -> MATLAB Function6/1(RxBytes)
  MATLAB Function7/1(Message) -> CAN Unpack7/1
  Read RX Buffer start at RXB0SIDH6/1 -> SPI Controller Transfer6/1
  CAN Unpack7/4 -> VDCInvRR/1
  CAN Unpack8/4 -> TInvRR/1
